simulink model "SPHERES_lyapnov_model_pulse_modulation"  (R2017b)
settings: Solver=ode4  StartTime=0.0  StopTime=349.99  FixedStep=0.05  RelTol=1e-3
InitFcn:
  | Mass = 4.16;
  | 
  | inertia(1,1) =  2.30E-2;  %kg m^2
  |             inertia(2,1) =  2.42E-2;
  |             inertia(3,1) =  2.14E-2;
  |             inertia(4,1) =  9.90E-05;
  |             inertia(5,1) = -2.95E-04;
  |             inertia(6,1) = -2.54E-05;
  | params.InertiaM = [inertia(1,1)  inertia(4,1)  inertia(5,1);...
  |                 inertia(4,1)  inertia(2,1)  inertia(6,1);...
  |                 inertia(5,1)  inertia(6,1)  inertia(3,1)];
  | 
  | params.Rorbit = 6378+400;
  | params.mu = 398600;
  | params.n = sqrt(params.mu/params.Rorbit^3); % angular velocity of the LRF
  | 
  | dx = 9.65E-2;
  | u_factor = 5;
  | ua = 0.12/u_factor;
  | min_pulse = 0.01;
  | 
  | HF = [1 1 0 0 0 0 -1 -1 0 0 0 0;...
  | 0 0 1 1 0 0 0 0 -1 -1 0 0;...
  | 0 0 0 0 1 1 0 0 0 0 -1 -1];
  | 
  | HM = [0 0 0 0 1 -1 0 0 0 0 -1 1;...
  |     1 -1 0 0 0 0 -1 1 0 0 0 0;...
  |     0 0 1 -1 0 0 0 0 -1 1 0 0]*dx;
  | H = [HF;HM];
  | 
  | uad_matrix = ua*eye(3)*dx;
  | 
  | % ref model variables
  | RM.v_pc = 0;
  | RM.v_sc = 0;
  | % xm0 = -10;
  | % ym0 = 10;
  | % zm0 = 10;
  | % RM.p_dot0 = [0.05, 0.05 -0.05];
  | % RM.angles0 = deg2rad([30, 30, -30]);
  | 
  | %%%%test block
  | xm0 = -10;
  | ym0 = 10;
  | zm0 = 10;
  | RM.p_dot0 = [0,0,0];
  | RM.angles0 = deg2rad([30,30,-30]);
  | % RM.angles0 = deg2rad([0,0,0]);
  | RM.s0_dot = [0,0,0];
  | RM.w0 = deg2rad([ 0,0,0]);
  | %%%%end test
  | RM.p0 = [xm0 ym0 zm0];
  | RM.q0 = flip(angle2quat(RM.angles0(1),RM.angles0(2),RM.angles0(3))); %MRPs
  | RM.s0 = RM.q0(1:3)/(1+RM.q0(4)); %verify MRP
  | % RM.s0_dot = [-0.0012708 -0.0005454   0.0037368];
  | % RM.w0 = deg2rad([ 6, -6, 6]);
  | % RM.K1 = diag([0.0258328125000000	0.0325984375000000	0.0258796875000000]);
  | % RM.K2 = diag([0.000250000000000000	0.000375000000000000	0.000257812500000000]);
  | %Perfect Fit
  | RM.K1 = diag([0.03440625, 0.031953125, 0.033859375]);
  | RM.K2 = 3.7e-4* diag([1, 1, 1]);
  | RM.K3 = diag([3.3105	4.6005	3.2305]);
  | RM.K4 = diag([0.4711	0.6936	0.4811]);
  | 
  | init_states = [RM.p0, RM.p_dot0, RM.s0, RM.w0];
  | % solve the lyapunov equation
  | Q1 = 5e4 * eye(6);
  | Q2 = 5e5 * eye(6);
  | A1m = [zeros(3,3),eye(3);-RM.K1,-RM.K2];
  | A2m = [zeros(3,3),eye(3);-RM.K3,-RM.K4];
  | P_p = lyap(A1m',Q1);
  | P_s = lyap(A2m',Q2);
  | K_p_T = [P_p(1:3,4:6),P_p(4:6,4:6)]';
  | K_s_T = [P_s(1:3,4:6),P_s(4:6,4:6)]';
settings Model: Creator=Reza  LastModifiedBy=Reza
settings DebuggingCC: SignalRangeChecking=error

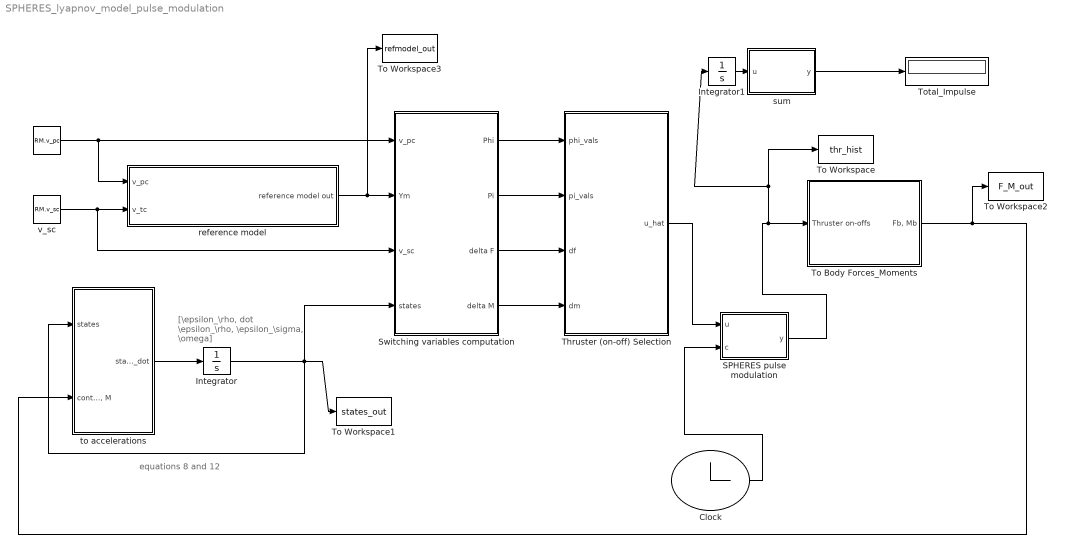
== system SPHERES_lyapnov_model_pulse_modulation ==
  note: equations 8 and 12
  note: [\epsilon_\rho, dot \epsilon_\rho, \epsilon_\sigma, \omega]
  " " : Constant  Value=RM.v_pc
  Clock : Clock
      settings: Decimation=4
  Integrator : Integrator  InitialCondition=init_states
  Integrator1 : Integrator
  "SPHERES pulse modulation " : MATLAB Function  TreatAsAtomicUnit=on
  Switching variables computation : Subsystem
  Thruster (on-off) Selection : MATLAB Function  TreatAsAtomicUnit=on
  To Body Forces_Moments : Subsystem
  To Workspace : ToWorkspace  VariableName=thr_hist  SaveFormat=Timeseries  SampleTime=-1
  To Workspace1 : ToWorkspace  VariableName=states_out  SaveFormat=Timeseries  SampleTime=-1
  To Workspace2 : ToWorkspace  VariableName=F_M_out  SaveFormat=Timeseries  SampleTime=-1
  To Workspace3 : ToWorkspace  VariableName=refmodel_out  SaveFormat=Timeseries  SampleTime=-1
  "Total_Impulse " : Display
  reference model : Subsystem
  sum : MATLAB Function  TreatAsAtomicUnit=on
  to accelerations : Subsystem
  "v_sc " : Constant  Value=RM.v_sc
  wires:
  reference model/1("reference model out ") -> To Workspace3/1, Switching variables computation/2(Ym)
  " "/1 -> Switching variables computation/1(v_pc), reference model/1(v_pc)
  "v_sc "/1 -> Switching variables computation/3(v_sc), reference model/2(v_tc)
  To Body Forces_Moments/1("Fb, Mb") -> To Workspace2/1, to accelerations/2("controls F, M")
  to accelerations/1(states_dot) -> Integrator/1
  Integrator/1 -> To Workspace1/1, Switching variables computation/4(states), to accelerations/1("states ")
  Integrator1/1 -> sum/1(u)
  sum/1(y) -> "Total_Impulse "/1
  Clock/1 -> "SPHERES pulse modulation "/2(c)
  Thruster (on-off) Selection/1(u_hat) -> "SPHERES pulse modulation "/1(u)
  "SPHERES pulse modulation "/1(y) -> Integrator1/1, To Workspace/1, To Body Forces_Moments/1(Thruster on-offs)
  Switching variables computation/1(Phi) -> Thruster (on-off) Selection/1(phi_vals)
  Switching variables computation/2(Pi) -> Thruster (on-off) Selection/2(pi_vals)
  Switching variables computation/3(delta F) -> Thruster (on-off) Selection/3(df)
  Switching variables computation/4(delta M) -> Thruster (on-off) Selection/4(dm)

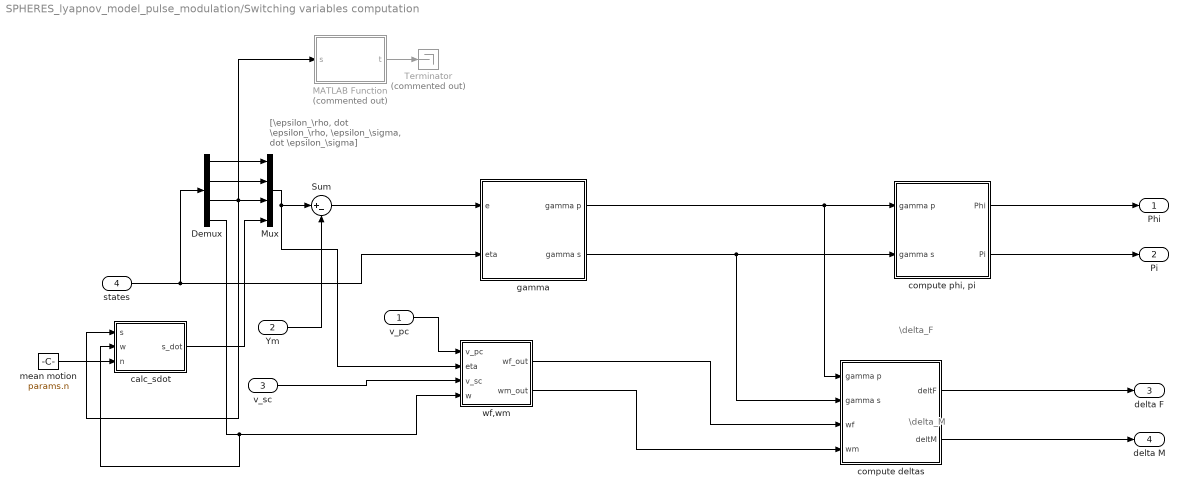
== system SPHERES_lyapnov_model_pulse_modulation/Switching variables computation ==
  note: \delta_F
  note: \delta_M
  note: [\epsilon_\rho, dot \epsilon_\rho, \epsilon_\sigma, dot \epsilon_\sigma]
  v_pc : Inport
  Ym : Inport  Port=2
  v_sc : Inport  Port=3
  states : Inport  Port=4
  Demux : Demux
  MATLAB Function : MATLAB Function  Commented=on  TreatAsAtomicUnit=on
  Mux : Mux
  Sum : Sum  Inputs=|+-
  Terminator : Terminator  Commented=on
  "calc_sdot " : MATLAB Function  TreatAsAtomicUnit=on
  compute deltas : Subsystem
  "compute phi, pi" : Subsystem
  gamma : Subsystem
  mean motion : Constant  Value=params.n
  wf,wm : Subsystem
  Phi : Outport
  Pi : Outport  Port=2
  delta F : Outport  Port=3
  delta M : Outport  Port=4
  wires:
  gamma/2(gamma s) -> "compute phi, pi"/2(gamma s), compute deltas/2(gamma s)
  gamma/1(gamma p) -> "compute phi, pi"/1(gamma p), compute deltas/1(gamma p)
  "compute phi, pi"/1(Phi) -> Phi/1
  "compute phi, pi"/2(Pi) -> Pi/1
  wf,wm/1(wf_out) -> compute deltas/3(wf)
  wf,wm/2(wm_out) -> compute deltas/4(wm)
  compute deltas/1(deltF) -> delta F/1
  compute deltas/2(deltM) -> delta M/1
  v_sc/1 -> wf,wm/3(v_sc)
  v_pc/1 -> wf,wm/1(v_pc)
  states/1 -> Demux/1, gamma/2(eta)
  Sum/1 -> gamma/1(e)
  Ym/1 -> Sum/2
  Mux/1 -> Sum/1, wf,wm/2(eta)
  Demux/4 -> "calc_sdot "/2(w), wf,wm/4(w)
  "calc_sdot "/1(s_dot) -> Mux/4
  Demux/3 -> MATLAB Function/1(s), "calc_sdot "/1(s), Mux/3
  Demux/2 -> Mux/2
  Demux/1 -> Mux/1
  mean motion/1 -> "calc_sdot "/3(n)
  MATLAB Function/1(t) -> Terminator/1

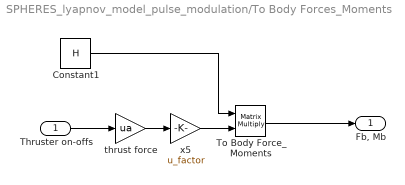
== system SPHERES_lyapnov_model_pulse_modulation/To Body Forces_Moments ==
  Thruster on-offs : Inport
  Constant1 : Constant  Value=H
  To Body Force_Moments : Product  Multiplication=Matrix(*)
  thrust force : Gain  Gain=ua
  "x5 " : Gain  Gain=u_factor
  "Fb, Mb" : Outport
  wires:
  Constant1/1 -> To Body Force_Moments/1
  To Body Force_Moments/1 -> "Fb, Mb"/1
  Thruster on-offs/1 -> thrust force/1
  "x5 "/1 -> To Body Force_Moments/2
  thrust force/1 -> "x5 "/1

== system SPHERES_lyapnov_model_pulse_modulation/reference model ==
  note: \sigma_m
  note: \rho_m
  note: dot \rho_m
  note: dot \sigma_m
  v_pc : Inport
  v_tc : Inport  Port=2
  Mux : Mux
  reference model - rotational : Subsystem
  "reference model - translational " : Subsystem
  "reference model out " : Outport
  wires:
  v_tc/1 -> reference model - rotational/1(v_tc)
  v_pc/1 -> "reference model - translational "/1(v_pc)
  Mux/1 -> "reference model out "/1
  "reference model - translational "/1("Yp_model ") -> Mux/1
  "reference model - translational "/2("pdot_model ") -> Mux/2
  reference model - rotational/1("Yt_model ") -> Mux/3
  reference model - rotational/2("t dot_model ") -> Mux/4

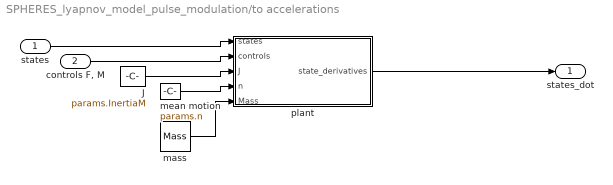
== system SPHERES_lyapnov_model_pulse_modulation/to accelerations ==
  "states " : Inport
  "controls F, M" : Inport  Port=2
  J : Constant  Value=params.InertiaM
  "mass " : Constant  Value=Mass
  mean motion : Constant  Value=params.n
  plant : MATLAB Function  TreatAsAtomicUnit=on
  states_dot : Outport
  wires:
  "states "/1 -> plant/1(states)
  "controls F, M"/1 -> plant/2(controls)
  J/1 -> plant/3(J)
  plant/1(state_derivatives) -> states_dot/1
  mean motion/1 -> plant/4(n)
  "mass "/1 -> plant/5(Mass)

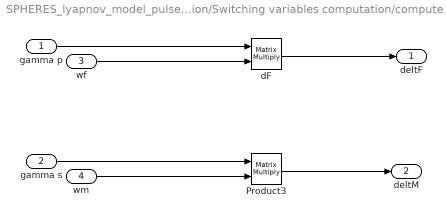
== system SPHERES_lyapnov_model_pulse_modulation/Switching variables computation/compute deltas ==
  gamma p : Inport
  gamma s : Inport  Port=2
  wf : Inport  Port=3
  wm : Inport  Port=4
  Product3 : Product  Multiplication=Matrix(*)
  dF : Product  Multiplication=Matrix(*)
  deltF : Outport
  deltM : Outport  Port=2
  wires:
  dF/1 -> deltF/1
  wf/1 -> dF/2
  wm/1 -> Product3/2
  Product3/1 -> deltM/1
  gamma p/1 -> dF/1
  gamma s/1 -> Product3/1

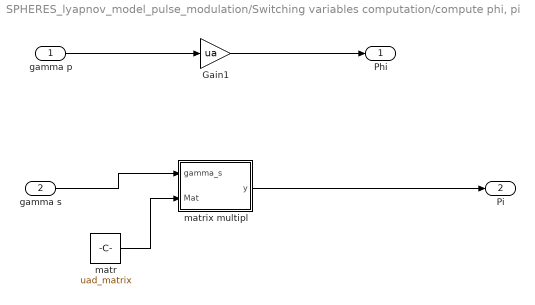
== system SPHERES_lyapnov_model_pulse_modulation/Switching variables computation/compute phi, pi ==
  gamma p : Inport
  gamma s : Inport  Port=2
  Gain1 : Gain  Gain=ua
  matr : Constant  Value=uad_matrix
  matrix multipl : MATLAB Function  TreatAsAtomicUnit=on
  Phi : Outport
  Pi : Outport  Port=2
  wires:
  Gain1/1 -> Phi/1
  gamma p/1 -> Gain1/1
  matr/1 -> matrix multipl/2(Mat)
  gamma s/1 -> matrix multipl/1(gamma_s)
  matrix multipl/1(y) -> Pi/1

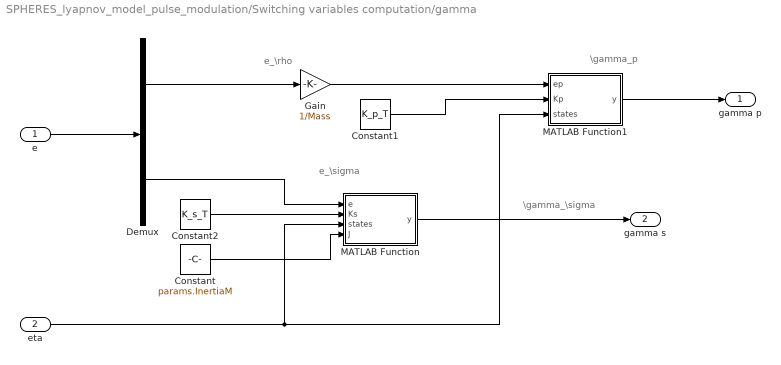
== system SPHERES_lyapnov_model_pulse_modulation/Switching variables computation/gamma ==
  note: \gamma_p
  note: e_\rho
  note: e_\sigma
  note: \gamma_\sigma
  e : Inport
  eta : Inport  Port=2
  Constant : Constant  Value=params.InertiaM
  Constant1 : Constant  Value=K_p_T
  Constant2 : Constant  Value=K_s_T
  Demux : Demux  Outputs=2
  Gain : Gain  Gain=1/Mass
  MATLAB Function : MATLAB Function  TreatAsAtomicUnit=on
  MATLAB Function1 : MATLAB Function  TreatAsAtomicUnit=on
  gamma p : Outport
  gamma s : Outport  Port=2
  wires:
  e/1 -> Demux/1
  Demux/1 -> Gain/1
  Constant2/1 -> MATLAB Function/2(Ks)
  eta/1 -> MATLAB Function/3(states), MATLAB Function1/3(states)
  Constant1/1 -> MATLAB Function1/2(Kp)
  MATLAB Function/1(y) -> gamma s/1
  MATLAB Function1/1(y) -> gamma p/1
  Gain/1 -> MATLAB Function1/1(ep)
  Demux/2 -> MATLAB Function/1(e)
  Constant/1 -> MATLAB Function/4(J)

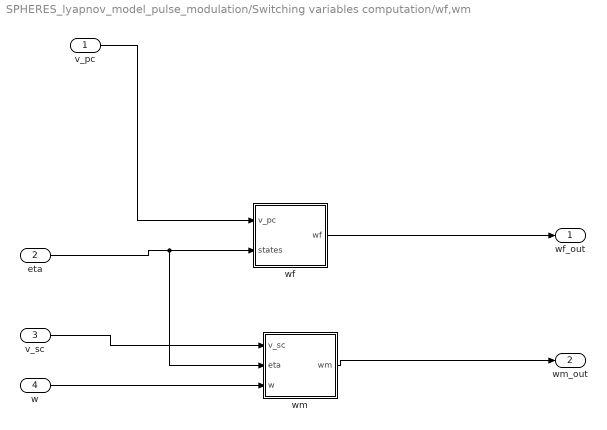
== system SPHERES_lyapnov_model_pulse_modulation/Switching variables computation/wf,wm ==
  v_pc : Inport
  eta : Inport  Port=2
  v_sc : Inport  Port=3
  w : Inport  Port=4
  wf : Subsystem
  wm : Subsystem
  wf_out : Outport
  wm_out : Outport  Port=2
  wires:
  eta/1 -> wm/2(eta), wf/2(states)
  v_pc/1 -> wf/1(v_pc)
  v_sc/1 -> wm/1(v_sc)
  wf/1(wf) -> wf_out/1
  wm/1(wm) -> wm_out/1
  w/1 -> wm/3(w)

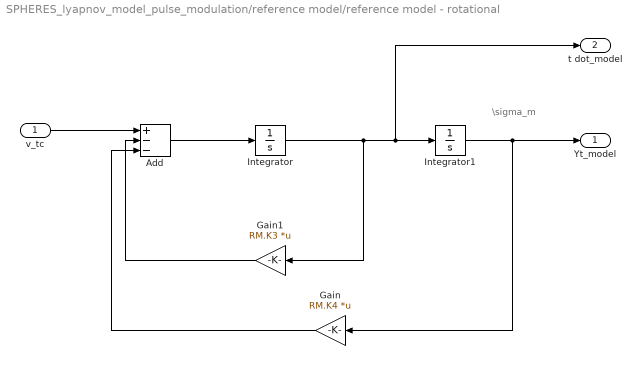
== system SPHERES_lyapnov_model_pulse_modulation/reference model/reference model - rotational ==
  note: \sigma_m
  v_tc : Inport
  Add : Sum  Inputs=+--
  Gain : Gain  Gain=RM.K4  Multiplication=Matrix(K*u)
  Gain1 : Gain  Gain=RM.K3  Multiplication=Matrix(K*u)
  Integrator : Integrator  InitialCondition=RM.s0_dot
  Integrator1 : Integrator  InitialCondition=RM.s0
  "Yt_model " : Outport
  "t dot_model " : Outport  Port=2
  wires:
  v_tc/1 -> Add/1
  Integrator1/1 -> "Yt_model "/1, Gain/1
  Gain1/1 -> Add/2
  Gain/1 -> Add/3
  Integrator/1 -> Gain1/1, "t dot_model "/1, Integrator1/1
  Add/1 -> Integrator/1

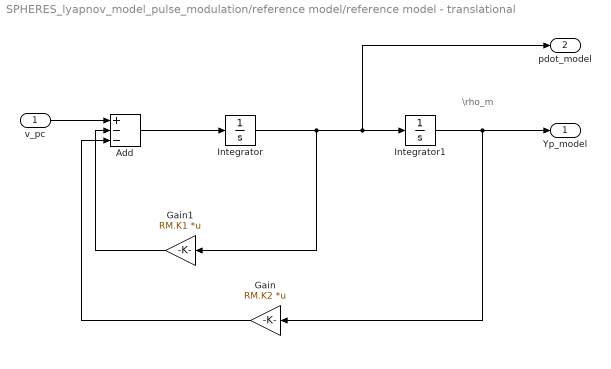
== system SPHERES_lyapnov_model_pulse_modulation/reference model/reference model - translational  ==
  note: \rho_m
  v_pc : Inport
  Add : Sum  Inputs=+--
  Gain : Gain  Gain=RM.K2  Multiplication=Matrix(K*u)
  Gain1 : Gain  Gain=RM.K1  Multiplication=Matrix(K*u)
  Integrator : Integrator  InitialCondition=RM.p_dot0
  Integrator1 : Integrator  InitialCondition=RM.p0
  "Yp_model " : Outport
  "pdot_model " : Outport  Port=2
  wires:
  v_pc/1 -> Add/1
  Integrator1/1 -> "Yp_model "/1, Gain/1
  Gain1/1 -> Add/2
  Gain/1 -> Add/3
  Add/1 -> Integrator/1
  Integrator/1 -> Gain1/1, "pdot_model "/1, Integrator1/1

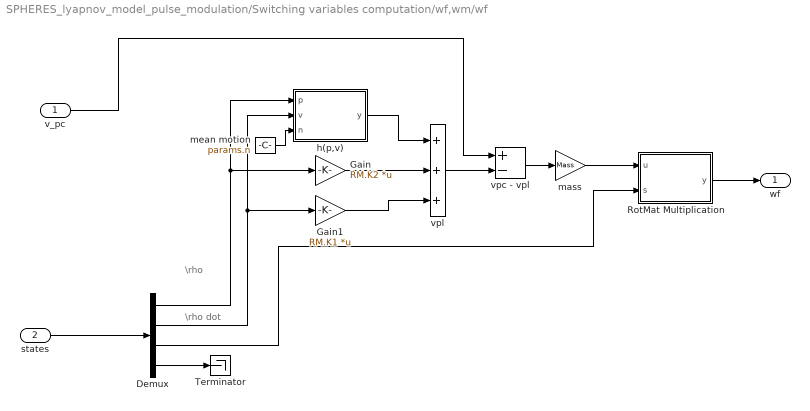
== system SPHERES_lyapnov_model_pulse_modulation/Switching variables computation/wf,wm/wf ==
  note: \rho dot
  note: \rho
  v_pc : Inport
  states : Inport  Port=2
  Demux : Demux
  Gain : Gain  Gain=RM.K2  Multiplication=Matrix(K*u)
  Gain1 : Gain  Gain=RM.K1  Multiplication=Matrix(K*u)
  "RotMat Multiplication " : MATLAB Function  TreatAsAtomicUnit=on
  Terminator : Terminator
  h(p,v) : MATLAB Function  TreatAsAtomicUnit=on
  "mass " : Gain  Gain=Mass
  mean motion : Constant  Value=params.n
  "vpc - vpl " : Sum  Inputs=+-
  vpl : Sum  Inputs=+++
  wf : Outport
  wires:
  states/1 -> Demux/1
  Gain/1 -> vpl/2
  Gain1/1 -> vpl/3
  v_pc/1 -> "vpc - vpl "/1
  vpl/1 -> "vpc - vpl "/2
  "vpc - vpl "/1 -> "mass "/1
  "mass "/1 -> "RotMat Multiplication "/1(u)
  "RotMat Multiplication "/1(y) -> wf/1
  Demux/2 -> Gain1/1, h(p,v)/2(v)
  Demux/1 -> Gain/1, h(p,v)/1(p)
  h(p,v)/1(y) -> vpl/1
  Demux/3 -> "RotMat Multiplication "/2(s)
  Demux/4 -> Terminator/1
  mean motion/1 -> h(p,v)/3(n)

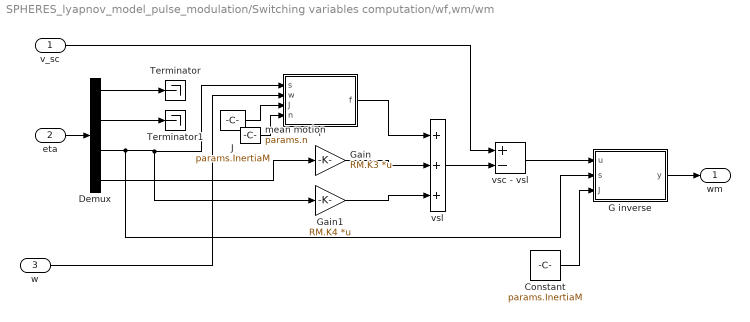
== system SPHERES_lyapnov_model_pulse_modulation/Switching variables computation/wf,wm/wm ==
  v_sc : Inport
  eta : Inport  Port=2
  w : Inport  Port=3
  Constant : Constant  Value=params.InertiaM
  Demux : Demux
  "G inverse " : MATLAB Function  TreatAsAtomicUnit=on
  Gain : Gain  Gain=RM.K3  Multiplication=Matrix(K*u)
  Gain1 : Gain  Gain=RM.K4  Multiplication=Matrix(K*u)
  J : Constant  Value=params.InertiaM
  Terminator : Terminator
  Terminator1 : Terminator
  f : MATLAB Function  TreatAsAtomicUnit=on
  mean motion : Constant  Value=params.n
  "vsc - vsl " : Sum  Inputs=+-
  vsl : Sum  Inputs=+++
  wm : Outport
  wires:
  "G inverse "/1(y) -> wm/1
  "vsc - vsl "/1 -> "G inverse "/1(u)
  vsl/1 -> "vsc - vsl "/2
  v_sc/1 -> "vsc - vsl "/1
  Gain1/1 -> vsl/3
  Gain/1 -> vsl/2
  eta/1 -> Demux/1
  f/1(f) -> vsl/1
  Demux/1 -> Terminator/1
  Demux/2 -> Terminator1/1
  Demux/4 -> Gain/1
  Demux/3 -> "G inverse "/2(s), f/1(s), Gain1/1
  Constant/1 -> "G inverse "/3(J)
  mean motion/1 -> f/4(n)
  J/1 -> f/3(J)
  w/1 -> f/2(w)

== matlab function SPHERES_lyapnov_model_pulse_modulation/Switching variables computation/calc_sdot  ==
  data: s input size=[3 1]; w input size=[3 1]; s_dot output; n input
function s_dot  = fcn(s, w, n)


%sigma (MRPs) derivatives
wL = [0;0;n];
s_dot = 0.25*C(s)*(w - SRotL(s) * wL);
%% test block
if( ~isequal(size(s),[3 1]) )
        error('wrong size for s at sdot')
end
%% 

function Mat = C(s)
Mat = (1 - s'*s)*eye(3) + 2*skew(s) + 2*(s*s');

function rotMat = SRotL(s) %rotation from LRF to SRF
s_tilde = skew(s);
rotMat = eye(3) + (8*s_tilde^2  - 4*(1-s'*s)* s_tilde )/(1 + s'*s)^2;

function s_tilde = skew(s)
s_tilde = [0, -s(3), s(2); s(3), 0, -s(1); -s(2), s(1), 0];

== matlab function SPHERES_lyapnov_model_pulse_modulation/Switching variables computation/wf,wm/wm/f ==
  data: s input size=[3 1]; f output; w input size=[3 1]; J input; n input
function f  = fcn(s, w, J, n)

%% test block
if( ~isequal(size(s),[3 1]) )
        error('wrong size for s at f')
end
%% 
%sigma (MRPs) derivatives
wL = [0;0;n];
s_dot = 0.25*C(s)*(w - SRotL(s) * wL);


%% calculate f

f = 0.25*(C_dot(s,s_dot)*(w - SRotL(s)*wL) + ...
    C(s)*(  ( J\(skew(w)*(J*w)) ) - R_dot(s,s_dot)*wL));




function Mat = C(s)
Mat = (1 - s'*s)*eye(3) + 2*skew(s) + 2*(s*s');

function rotMat = SRotL(s) %rotation from LRF to SRF
s_tilde = skew(s);
rotMat = eye(3) + (8*s_tilde^2  - 4*(1-s'*s)* s_tilde )/(1 + s'*s)^2;

function s_tilde = skew(s)
s_tilde = [0, -s(3), s(2); s(3), 0, -s(1); -s(2), s(1), 0];

% function r = G(s,J)
% r = J\(0.25*C(s));

function res = C_dot(svec,svec_dot)
res = (- 2*svec_dot'*svec)*eye(3) + 2*skew(svec_dot) + 2*(svec_dot*svec') + 2*(svec*svec_dot');

function R_dot = R_dot(s,s_dot)
%R_DOT
%    R_DOT = R_DOT(S1,S2,S3,SD1,SD2,SD3)

%    This function was generated by the Symbolic Math Toolbox version 8.0.
%    01-Apr-2018 22:13:05
s1 = s(1);
s2 = s(2);
s3 = s(3);
sd1 = s_dot(1);
sd2 = s_dot(2);
sd3 = s_dot(3);

%Version: 1.1
t2 = s2.^2;
t3 = s3.^2;
t4 = s1.^2;
t5 = t2+t3+t4+1.0;
t6 = 1.0./t5.^2;
t7 = t4.*4.0;
t8 = t2.*4.0;
t9 = t3.*4.0;
t10 = t7+t8+t9-4.0;
t11 = s1.*sd1.*2.0;
t12 = s2.*sd2.*2.0;
t13 = s3.*sd3.*2.0;
t14 = t11+t12+t13;
t15 = 1.0./t5.^3;
t16 = s1.*sd1.*8.0;
t17 = s2.*sd2.*8.0;
t18 = s3.*sd3.*8.0;
t19 = t16+t17+t18;
t20 = s1.*sd2.*8.0;
t21 = s2.*sd1.*8.0;
t22 = s1.*s2.*8.0;
t23 = s3.*sd3.*1.6e1;
t24 = t3.*8.0;
t25 = s2.*t19;
t26 = s1.*sd3.*8.0;
t27 = s3.*sd1.*8.0;
t28 = sd2.*t10;
t29 = s1.*s3.*8.0;
t30 = s2.*t10;
t31 = s2.*sd3.*8.0;
t32 = s3.*sd2.*8.0;
t33 = s2.*s3.*8.0;
t34 = s1.*sd1.*1.6e1;
t35 = s2.*sd2.*1.6e1;
t36 = t4.*8.0;
t37 = t2.*8.0;
R_dot = reshape([-t6.*(t23+t35)+t14.*t15.*(t24+t37).*2.0,t6.*(t20+t21+s3.*t19+sd3.*t10)-t14.*t15.*(t22+s3.*t10).*2.0,-t6.*(t25-t26-t27+t28)-t14.*t15.*(t29-t30).*2.0,t6.*(t20+t21-s3.*t19-sd3.*t10)-t14.*t15.*(t22-s3.*t10).*2.0,-t6.*(t23+t34)+t14.*t15.*(t24+t36).*2.0,t6.*(t31+t32+s1.*t19+sd1.*t10)-t14.*t15.*(t33+s1.*t10).*2.0,t6.*(t25+t26+t27+t28)-t14.*t15.*(t29+t30).*2.0,t6.*(t31+t32-s1.*t19-sd1.*t10)-t14.*t15.*(t33-s1.*t10).*2.0,-t6.*(t34+t35)+t14.*t15.*(t36+t37).*2.0],[3,3]);

== matlab function SPHERES_lyapnov_model_pulse_modulation/to accelerations/plant ==
  data: states input size=[12 1]; state_derivatives output; controls input size=6; J input; n input; Mass input
function state_derivatives  = fcn(states, controls, J, n, Mass)

p = states(1:3);
v = states(4:6);
s = states(7:9);
w = states(10:12);
%% test block
if( ~isequal(size(s),[3 1]) )
        error('wrong size for s')
end
%% 
FB = controls(1:3);
FL = SRotL(-s)*FB;
MB = controls([4:6]);


deriv_1 = v;
% CW equations
deriv_2 = h(p,v,n) + FL/Mass;


%sigma (MRPs) derivatives
wL = [0;0;n];
deriv_3 = 0.25*C(s)*(w - SRotL(s) * wL);
s_dot = deriv_3;

%omega (w) derivative
deriv_4 = J\(-1*skew(w)*(J*w) + MB);
% deriv_4 = J\(MB - cross(w, J*w));
w_dot = deriv_4;

% if(sum (deriv_4(:) - deriv_42(:)) > 1e-12) 
% error('wrong w_dot calculation'),
% end

%collect
state_derivatives = [ deriv_1;deriv_2;deriv_3;deriv_4];

%% calculate f

% s_deriv_deriv = 0.25*(C_dot(s,s_dot)*(w - SRotL(s)*wL) + ...
%     C(s)*(w_dot - R_dot(s,s_dot)*wL));
% f = 0.25*(C_dot(s,s_dot)*(w - SRotL(s)*wL) + ...
%     C(s)*(  ( J\(skew(w)*(J*w)) ) - R_dot(s,s_dot)*wL));
% f2 = s_deriv_deriv - G(s,J)*MB;
% chk = abs(f2 - f);
% % 
% if( chk > 1e-5 ) error('wrong f calculation as much a'), end

function deriv = h(p,v,n)
% deriv =  [((2*mu_/norm_R_^3 + H_^2/norm_R_^4)*x1 - 2*RdotV_/norm_R_^4*H_*x2 + 2*H_/norm_R_^2*v2);
%             (-(mu_/norm_R_^3 - H_^2/norm_R_^4)*x2 + 2*RdotV_/norm_R_^4*H_*x1 - 2*H_/norm_R_^2*v1);
%             (-mu_/norm_R_^3*x3)];
            
deriv = [3*n^2*p(1) + 2*n*v(2);...
    -2*n*v(1);...
    -n^2*p(3)];

function Mat = C(s)
Mat = (1 - s'*s)*eye(3) + 2*skew(s) + 2*(s*s');

function rotMat = SRotL(s) %rotation from LRF to SRF
s_tilde = skew(s);
rotMat = eye(3) + (8*s_tilde^2  - 4*(1-s'*s)* s_tilde )/(1 + s'*s)^2;

function s_tilde = skew(s)
s_tilde = [0, -s(3), s(2); s(3), 0, -s(1); -s(2), s(1), 0];

function r = G(s,J)
r = J\(0.25*C(s));

function res = C_dot(svec,svec_dot)
res = (- 2*svec_dot'*svec)*eye(3) + 2*skew(svec_dot) + 2*(svec_dot*svec') + 2*(svec*svec_dot');

function R_dot = R_dot(s,s_dot)
%R_DOT
%    R_DOT = R_DOT(S1,S2,S3,SD1,SD2,SD3)

%    This function was generated by the Symbolic Math Toolbox version 8.0.
%    01-Apr-2018 22:13:05
s1 = s(1);
s2 = s(2);
s3 = s(3);
sd1 = s_dot(1);
sd2 = s_dot(2);
sd3 = s_dot(3);

%Version: 1.1
t2 = s2.^2;
t3 = s3.^2;
t4 = s1.^2;
t5 = t2+t3+t4+1.0;
t6 = 1.0./t5.^2;
t7 = t4.*4.0;
t8 = t2.*4.0;
t9 = t3.*4.0;
t10 = t7+t8+t9-4.0;
t11 = s1.*sd1.*2.0;
t12 = s2.*sd2.*2.0;
t13 = s3.*sd3.*2.0;
t14 = t11+t12+t13;
t15 = 1.0./t5.^3;
t16 = s1.*sd1.*8.0;
t17 = s2.*sd2.*8.0;
t18 = s3.*sd3.*8.0;
t19 = t16+t17+t18;
t20 = s1.*sd2.*8.0;
t21 = s2.*sd1.*8.0;
t22 = s1.*s2.*8.0;
t23 = s3.*sd3.*1.6e1;
t24 = t3.*8.0;
t25 = s2.*t19;
t26 = s1.*sd3.*8.0;
t27 = s3.*sd1.*8.0;
t28 = sd2.*t10;
t29 = s1.*s3.*8.0;
t30 = s2.*t10;
t31 = s2.*sd3.*8.0;
t32 = s3.*sd2.*8.0;
t33 = s2.*s3.*8.0;
t34 = s1.*sd1.*1.6e1;
t35 = s2.*sd2.*1.6e1;
t36 = t4.*8.0;
t37 = t2.*8.0;
R_dot = reshape([-t6.*(t23+t35)+t14.*t15.*(t24+t37).*2.0,t6.*(t20+t21+s3.*t19+sd3.*t10)-t14.*t15.*(t22+s3.*t10).*2.0,-t6.*(t25-t26-t27+t28)-t14.*t15.*(t29-t30).*2.0,t6.*(t20+t21-s3.*t19-sd3.*t10)-t14.*t15.*(t22-s3.*t10).*2.0,-t6.*(t23+t34)+t14.*t15.*(t24+t36).*2.0,t6.*(t31+t32+s1.*t19+sd1.*t10)-t14.*t15.*(t33+s1.*t10).*2.0,t6.*(t25+t26+t27+t28)-t14.*t15.*(t29+t30).*2.0,t6.*(t31+t32-s1.*t19-sd1.*t10)-t14.*t15.*(t33-s1.*t10).*2.0,-t6.*(t34+t35)+t14.*t15.*(t36+t37).*2.0],[3,3]);

== matlab function SPHERES_lyapnov_model_pulse_modulation/Switching variables computation/wf,wm/wf/RotMat Multiplication  ==
  data: u input size=[3,1]; y output; s input size=3
function y = fcn(u, s)

%% test block
if( ~isequal(size(s),[3 1]) )
        error('wrong size for s at RotMat wf')
end
%% 
y = SRotL(s)*u;



function rotMat = SRotL(s) %rotation from LRF to SRF
s_tilde = skew(s);
rotMat = eye(3) + (8*s_tilde^2  - 4*(1-s'*s)* s_tilde )/(1 + s'*s)^2;

function s_tilde = skew(s)
s_tilde = [0, -s(3), s(2); s(3), 0, -s(1); -s(2), s(1), 0];

== matlab function SPHERES_lyapnov_model_pulse_modulation/Switching variables computation/wf,wm/wf/h(p,v) ==
  data: p input size=3; y output size=3; v input size=3; n input
function y = fcn(p,v,n)

y = h(p,v,n);

function deriv = h(p,v,n)
deriv = [3*n^2*p(1) + 2*n*v(2);...
    -2*n*v(1);...
    -n^2*p(3)];

== matlab function SPHERES_lyapnov_model_pulse_modulation/Switching variables computation/gamma/MATLAB Function ==
  data: e input; y output size=[1,3]; Ks input; states input; J input
function y = fcn(e,Ks,states,J)

s = states(7:9);
Gmat = G(s,J);
y = e'*Ks*Gmat;

%% test block
if( ~isequal(size(s),[3 1]) )
        error('wrong size for s at gamma')
end
%% 


function r = G(s,J)

r = J\(0.25*C(s));

function Mat = C(s)
Mat = (1 - s'*s)*eye(3) + 2*skew(s) + 2*(s*s');

function s_tilde = skew(s)
s_tilde = [0, -s(3), s(2); s(3), 0, -s(1); -s(2), s(1), 0];

== matlab function SPHERES_lyapnov_model_pulse_modulation/Switching variables computation/gamma/MATLAB Function1 ==
  data: ep input; y output size=[1 3]; Kp input; states input
function y = fcn(ep,Kp,states)
s = states(7:9);
%% test block
if( ~isequal(size(s),[3 1]) )
        error('wrong size for s')
end
%% 

RotMats = SRotL(-s);
y = ep'*Kp*RotMats;

function rotMat = SRotL(s) %rotation from LRF to SRF
s_tilde = skew(s);
rotMat = eye(3) + (8*s_tilde^2  - 4*(1-s'*s)* s_tilde )/(1 + s'*s)^2;

function s_tilde = skew(s)
s_tilde = [0, -s(3), s(2); s(3), 0, -s(1); -s(2), s(1), 0];

== matlab function SPHERES_lyapnov_model_pulse_modulation/Thruster (on-off) Selection ==
  data: phi_vals input; u_hat output; pi_vals input size=[3,1]; df input; dm input
function u_hat = fcn(phi_vals, pi_vals, df, dm)
% %test

%% skips controlling ATTITUDE
% pi_vals = pi_vals*0;
% dm = dm*0;

%% skips controlling POSITION
% phi_vals = phi_vals*0;
% df = df*0;

% %end test

u_hat = zeros(12,1);
pi_vals = pi_vals';
Beta_p_T = fun_B_p_T(phi_vals);
Beta_s_T = fun_B_s_T(pi_vals);


    % should we check df + dm < 0 ?
if(df + dm < 0)
if( isNegative(df) && isPositive(dm))
    %initialize vectors
    phi_hat = zeros(1,3);
    phi_tilde = phi_vals;
    
%     while( Beta_p_T*u_hat - df - dm > 0)
    for jj = 1:length(phi_vals)
        [~,i_max_phi] = max(abs(phi_tilde));
        phi_hat(i_max_phi) = phi_vals(i_max_phi);
        phi_tilde(i_max_phi) = 0;
        Beta_p_T_hat = fun_B_p_T(phi_hat);
        u_hat = S(Beta_p_T_hat');
        if (Beta_p_T*u_hat - df - dm <= 0) 
            break
        end
    end

elseif( isPositive(df) && isNegative(dm))
    %initialize vectors
    pi_hat = zeros(1,3);
    pi_tilde = pi_vals;
    
    for jj = 1:length(pi_vals)
%     while( Beta_s_T*u_hat - df - dm > 0)
        [~,j_max_pi] = max(abs(pi_tilde));
        pi_hat(j_max_pi) = pi_vals(j_max_pi);
        pi_tilde(j_max_pi) = 0;
        Beta_s_T_hat = fun_B_s_T(pi_hat);
        u_hat = S(Beta_s_T_hat');
        
        if (Beta_s_T*u_hat - df - dm <= 0) 
            break
        end
        
    end
    
elseif( isNegative(df) && isNegative(dm))
    Beta_hat = zeros(1,12);
    id_match = Beta_p_T < 0 & Beta_s_T < 0;
    %solution 1
%     Beta_tilde = zeros(1,8);
%     Beta_tilde(id_match) = Beta_p_T(id_match) + Beta_s_T(id_match);
    %solution 2
    Beta_tilde = Beta_p_T + Beta_s_T;
    Beta_tilde(~id_match) = 0;
    
%     while((Beta_p_T + Beta_s_T)*u_hat - df - dm > 0)
    for jj = 1:6
    [~,id_h] = min(Beta_tilde); %most negative value
    Beta_hat(id_h) = Beta_tilde(id_h);
    Beta_tilde(id_h) = 0;
    u_hat = S(Beta_hat');
     if ((Beta_p_T + Beta_s_T)*u_hat - df - dm <= 0) 
            break
     end
    end
    
end
end
function switch_ = S(b)
switch_ = b*0;
switch_(b < 0) = 1;

function Beta_p_T = fun_B_p_T(phi_vals_)
Beta_p_T = phi_vals_([1,1,2,2,3,3,1,1,2,2,3,3]).*...
    [1,1,1,1,1,1,-1,-1,-1,-1,-1,-1];

function Beta_s_T = fun_B_s_T(pi_val_)
Beta_s_T = pi_val_([2,2,3,3,1,1,2,2,3,3,1,1]).*...
    [1,-1,1,-1,1,-1,-1,1,-1,1,-1,1];

function b = isPositive(val)
tol = 1e-15;
    b = val > -tol;


function b = isNegative(val)
tol = 1e-15;
    b = val < -tol;

== matlab function SPHERES_lyapnov_model_pulse_modulation/Switching variables computation/compute phi, pi/matrix multipl ==
  data: gamma_s input; y output; Mat input
function y = fcn(gamma_s, Mat)

y = Mat*gamma_s';

== matlab function SPHERES_lyapnov_model_pulse_modulation/Switching variables computation/wf,wm/wm/G inverse  ==
  data: u input; y output size=[3,1]; s input; J input
function y = fcn(u, s, J)

y = G(s,J)\u;
%% test block
if( ~isequal(size(s),[3 1]) )
        error('wrong size for s at Ginv')
end
%% 
function r = G(s,J)
r = J\(0.25*C(s));

function Mat = C(s)
Mat = (1 - s'*s)*eye(3) + 2*skew(s) + 2*(s*s');

function s_tilde = skew(s)
s_tilde = [0, -s(3), s(2); s(3), 0, -s(1); -s(2), s(1), 0];

== matlab function SPHERES_lyapnov_model_pulse_modulation/Switching variables computation/MATLAB Function ==
  data: s input; t output size=[3,1]
function t = fcn(s)

q = mrp2quat(s);

t = 2*asin(q(1:3));

== matlab function SPHERES_lyapnov_model_pulse_modulation/sum ==
  data: u input; y output
function y = fcn(u)

y = sum(u);

== matlab function SPHERES_lyapnov_model_pulse_modulation/SPHERES pulse modulation  ==
  settings: updateMethod=DISCRETE
  data: u input; y output; c input
function y = fcn(u,c)

% persistent q

% if isempty(q)
%     q = u;
% end
% 
% if rem(c,1) < 1e-3
%     % program the next 200 ms pulses
%     q = u;
% end

if rem(c,1) < 0.2
    y = u;
else
    y = 0*u;
end
